simulink model "amSSB1_WithHint"  (Simulink 8.3)
settings: Solver=ode45  StartTime=0.0  StopTime=1.5  RelTol=1e-3
undefined symbols (not defined in the file or in its folder): get
libraries: dsparch4 x4, dspspect3 x3, dspsnks4 x3
settings Model: Creator=gmessier  LastModifiedBy=maalmasr  ExtModeAutoUpdateStatusClock=off
settings DataIOCC: SignalLoggingName=sigsOut
settings OptimizationCC: ExpressionDepthLimit=2147483647  InitFltsAndDblsToZero=on
settings DebuggingCC: SaveWithParameterizedLinksMsg=none  SignalResolutionControl=TryResolveAllWithWarning  SolverPrmCheckMsg=none  MultiTaskDSMMsg=warning  MultiTaskCondExecSysMsg=none  FcnCallInpInsideContextMsg=UseLocalSettings
settings HardwareCC: TargetUnknown=on
settings RTWCC: IncludeERTFirstTime=on
settings GRTTargetCC: TargetFcnLib=ansi_tfl_tmw.mat  ModelReferenceCompliant=off  ParMdlRefBuildCompliant=off  CompOptLevelCompliant=off  ConcurrentExecutionCompliant=off  MatFileLogging=off

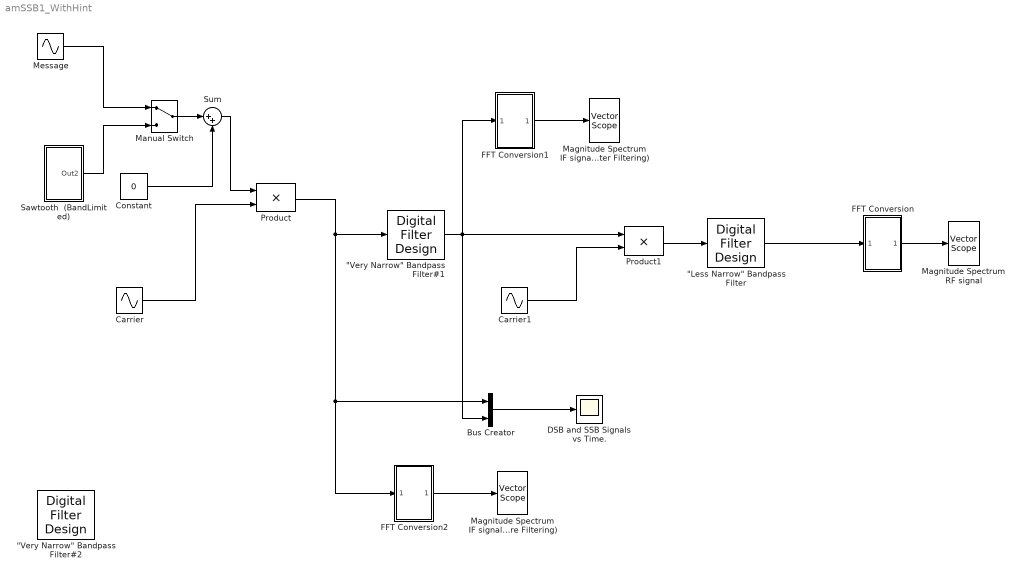
== system amSSB1_WithHint ==
  "\"Less Narrow\" Bandpass Filter" : dsparch4/Digital Filter Design  mwdsp_browser_bugfix_var=off
  "\"Very Narrow\" Bandpass Filter#1" : dsparch4/Digital Filter Design  mwdsp_browser_bugfix_var=off
  "\"Very Narrow\" Bandpass Filter#2" : dsparch4/Digital Filter Design  mwdsp_browser_bugfix_var=off
  Bus Creator : BusCreator  Inputs=2
  Carrier : Sin  Frequency=900*2*pi  SampleTime=1/16000
      settings: AttributesFormatString=Frequency = %<Frequency>\nAmplitude = %<Amplitude>
  Carrier1 : Sin  Frequency=4100*2*pi  SampleTime=1/16000
      settings: AttributesFormatString=Frequency = %<Frequency>
  Constant : Constant  Value=0
  DSB and SSB Signals vs Time. : Scope
      settings: TickLabels=on
  FFT Conversion : Subsystem
  FFT Conversion1 : Subsystem
  FFT Conversion2 : Subsystem
  Magnitude Spectrum IF signal (After Filtering) : dspsnks4/Vector Scope  ScopeProperties=off  Domain=Frequency  HorizSpan=1  DisplayProperties=off  AxisGrid=on  Memory=off  FrameNumber=on  AxisLegend=off  AxisZoom=off  OpenScopeAtSimStart=on  OpenScopeImmediately=off  FigPos=get(0,'defaultfigureposition')  AxisProperties=on  XUnits=Hertz  XRange=[0...Fs/2]  InheritXIncr=on  XIncr=1  XLabel=Time  XLimit=Auto  XMin=0  XMax=1  XStart=0  YUnits=Magnitude  YLabel=Amplitude  LineProperties=off  XAxisParamsVer=6.9
      settings: YMin=6.26793647632203e-007  YMax=0.195388027288579
  Magnitude Spectrum IF signal (Before Filtering) : dspsnks4/Vector Scope  ScopeProperties=off  Domain=Frequency  HorizSpan=1  DisplayProperties=off  AxisGrid=on  Memory=off  FrameNumber=on  AxisLegend=off  AxisZoom=off  OpenScopeAtSimStart=on  OpenScopeImmediately=off  FigPos=get(0,'defaultfigureposition')  AxisProperties=on  XUnits=Hertz  XRange=[0...Fs/2]  InheritXIncr=on  XIncr=1  XLabel=Time  XLimit=Auto  XMin=0  XMax=1  XStart=0  YUnits=Magnitude  YLabel=Amplitude  LineProperties=off  XAxisParamsVer=6.9
      settings: YMin=6.26793647632203e-007  YMax=0.195388027288579
  Magnitude Spectrum RF signal : dspsnks4/Vector Scope  ScopeProperties=off  Domain=Frequency  HorizSpan=1  DisplayProperties=off  AxisGrid=on  Memory=off  FrameNumber=on  AxisLegend=off  AxisZoom=off  OpenScopeAtSimStart=on  OpenScopeImmediately=off  FigPos=get(0,'defaultfigureposition')  AxisProperties=on  XUnits=Hertz  XRange=[0...Fs/2]  InheritXIncr=on  XIncr=1  XLabel=Time  XLimit=Auto  XMin=0  XMax=1  XStart=0  YUnits=Magnitude  YLabel=Amplitude  LineProperties=off  XAxisParamsVer=6.9
      settings: YMin=5.94344958967451e-005  YMax=0.0942727049852764
  Manual Switch : ManualSwitch
  Message : Sin  Amplitude=0.8  Frequency=300*2*pi  SampleTime=1/16000
      settings: AttributesFormatString=Frequency = %<Frequency>\nm = %<Amplitude>
  Product : Product  OutDataTypeStr=Inherit: Same as first input
  Product1 : Product  SaturateOnIntegerOverflow=on  OutDataTypeStr=Inherit: Same as first input
  Sawtooth  (BandLimited) : Subsystem
  Sum : Sum  Inputs=|++  SaturateOnIntegerOverflow=on
  wires:
  Carrier/1 -> Product/2
  Constant/1 -> Sum/2
  Sum/1 -> Product/1
  Bus Creator/1 -> DSB and SSB Signals vs Time./1
  Product/1 -> "\"Very Narrow\" Bandpass Filter#1"/1, Bus Creator/1, FFT Conversion2/1(In1)
  Carrier1/1 -> Product1/2
  FFT Conversion/1(Out1) -> Magnitude Spectrum RF signal/1
  FFT Conversion1/1(Out1) -> Magnitude Spectrum IF signal (After Filtering)/1
  Product1/1 -> "\"Less Narrow\" Bandpass Filter"/1
  "\"Less Narrow\" Bandpass Filter"/1 -> FFT Conversion/1(In1)
  "\"Very Narrow\" Bandpass Filter#1"/1 -> FFT Conversion1/1(In1), Product1/1, Bus Creator/2
  Manual Switch/1 -> Sum/1
  Message/1 -> Manual Switch/1
  Sawtooth  (BandLimited)/1(Out2) -> Manual Switch/2
  FFT Conversion2/1(Out1) -> Magnitude Spectrum IF signal (Before Filtering)/1

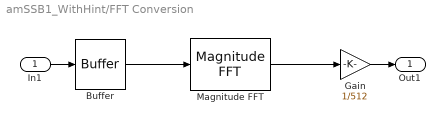
== system amSSB1_WithHint/FFT Conversion ==
  In1 : Inport
  Buffer : Buffer  N=512  TreatMby1Signals=One channel
  Gain : Gain  Gain=1/512  SaturateOnIntegerOverflow=on  OutDataTypeStr=Inherit: Same as input  ParamDataTypeStr=Inherit: Same as input
  Magnitude FFT : dspspect3/Magnitude FFT  mag_or_magsq=Magnitude  FFTImplementation=Auto  fftLenInherit=on  fftsize=256  WrapInput=on
  Out1 : Outport
  wires:
  Buffer/1 -> Magnitude FFT/1
  Magnitude FFT/1 -> Gain/1
  In1/1 -> Buffer/1
  Gain/1 -> Out1/1

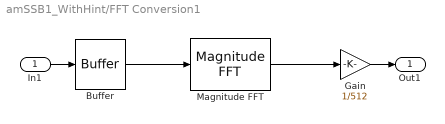
== system amSSB1_WithHint/FFT Conversion1 ==
  In1 : Inport
  Buffer : Buffer  N=512  TreatMby1Signals=One channel
  Gain : Gain  Gain=1/512  SaturateOnIntegerOverflow=on  OutDataTypeStr=Inherit: Same as input  ParamDataTypeStr=Inherit: Same as input
  Magnitude FFT : dspspect3/Magnitude FFT  mag_or_magsq=Magnitude  FFTImplementation=Auto  fftLenInherit=on  fftsize=256  WrapInput=on
  Out1 : Outport
  wires:
  Buffer/1 -> Magnitude FFT/1
  Magnitude FFT/1 -> Gain/1
  In1/1 -> Buffer/1
  Gain/1 -> Out1/1

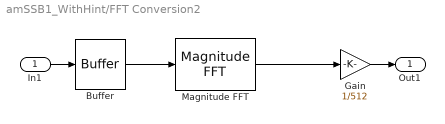
== system amSSB1_WithHint/FFT Conversion2 ==
  In1 : Inport
  Buffer : Buffer  N=512  TreatMby1Signals=One channel
  Gain : Gain  Gain=1/512  SaturateOnIntegerOverflow=on  OutDataTypeStr=Inherit: Same as input  ParamDataTypeStr=Inherit: Same as input
  Magnitude FFT : dspspect3/Magnitude FFT  mag_or_magsq=Magnitude  FFTImplementation=Auto  fftLenInherit=on  fftsize=256  WrapInput=on
  Out1 : Outport
  wires:
  Buffer/1 -> Magnitude FFT/1
  Magnitude FFT/1 -> Gain/1
  In1/1 -> Buffer/1
  Gain/1 -> Out1/1

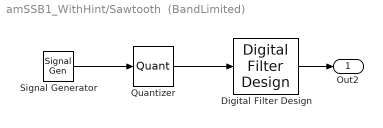
== system amSSB1_WithHint/Sawtooth  (BandLimited) ==
  Digital Filter Design : dsparch4/Digital Filter Design  mwdsp_browser_bugfix_var=off
  Quantizer : Quantizer  QuantizationInterval=0.05  SampleTime=1/16000
  Signal Generator : SignalGenerator  WaveForm=sawtooth  Frequency=125
  Out2 : Outport
  wires:
  Signal Generator/1 -> Quantizer/1
  Digital Filter Design/1 -> Out2/1
  Quantizer/1 -> Digital Filter Design/1
